simulink model "Electrical_System_2018b_obfs"  (R2019b)
settings: Solver=VariableStepAuto  StartTime=0.0  StopTime=5  RelTol=1e-3  AbsTol=1e-3  EnableMultiTasking=on
InitFcn:
  | Steady_State_Initialisation;
StopFcn:
  | %sscexplore(simlog);
  | %Logging
undefined symbols (not defined in the file): abrlhklxvp, aexgmhuedq, afmfmjnutg, afpphrjpnc, ahuxbyvruc, alarvljztt, amxnyqmnuw, aodrlwvqie, aolhmuplyq, aqpmguuqkg, auesgwirzl, aurophlnng, awamelrhru, ayfhvxflxn, azxkacuhqc, babszerikg, bawhdqanwq, bevoqecvei, bltjvqbchx, bmqsuewujl, bsmyqjfgnf, btvjbsmnve, bywgxqeadw, bziaduxaer, bzmcmdqocb, bzsvyvetat, ccsjnrbsih, cdvenygxwh, cedkrnslhx, cjheorclzs, cjrdshrtqx, ckhavyhcza, ckxewznhlz, cmrcgyiplk, conenicnws, cqkejbgjnn, csfnuwymhe, cunupkhwbh, cwzfvzuxxh, dcadmadufn, dcfponivnv, ddtrqjrhjn, dfhoxvkqas, dfrhtcwpne, dfvomcagjv, djijwylxea, dnmeqksrrm, dnzewbdkaa, dsqcykyxav, dtswwlttmm, ecumpidjtv, edegaywrct, ejjjsmnejc, eknqnehjdz, emvdetzouf, esxbqkbahr, etnkkbreiq, eunoiiiirw, ewewcuedir, fatkfxdhtc ... (+386)
libraries: fl_lib x802, ee_lib x362, fl_ps_legacy_lib x160, nesl_utility x85
(part 7 of 26)

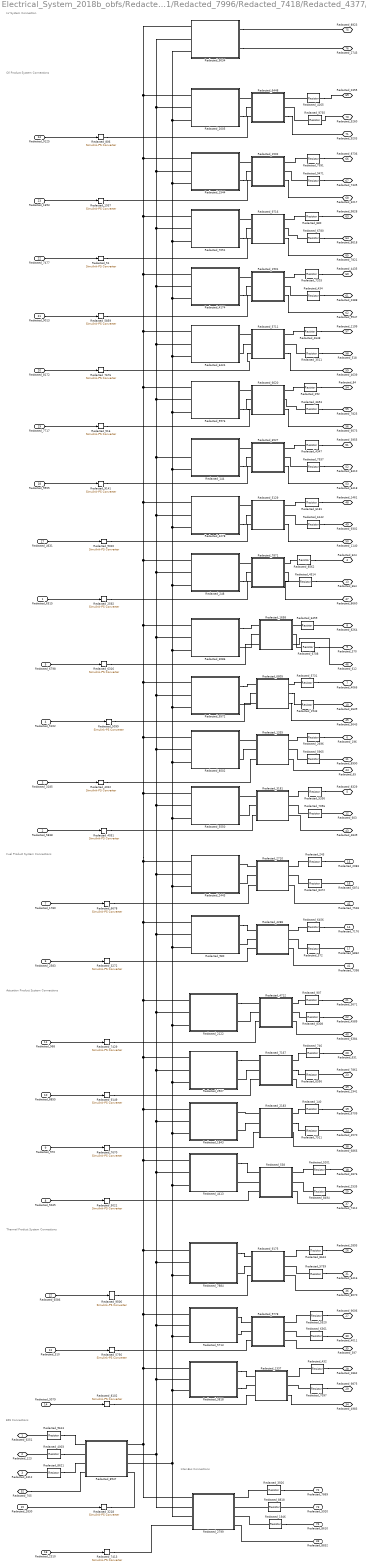
== system Electrical_System_2018b_obfs/Redacted_1221/Redacted_7996/Redacted_7418/Redacted_4377/Redacted_6082 ==
  note: LV System Connection
  note: Oil Product System Connections
  note: Fuel Product System Connections
  note: Actuation Product System Connections
  note: Thermal Product System Connections
  note: Inter-Bus Connections
  note: ESS Connections
  Redacted_6515 : Inport
  Redacted_5838 : Inport  Port=2
  Redacted_3185 : Inport  Port=3
  Redacted_5102 : Inport  Port=4
  Redacted_6798 : Inport  Port=5
  Redacted_2583 : Inport  Port=6
  Redacted_1780 : Inport  Port=7
  Redacted_5045 : Inport  Port=8
  Redacted_970 : Inport  Port=9
  Redacted_8855 : Inport  Port=10
  Redacted_968 : Inport  Port=11
  Redacted_6586 : Inport  Port=12
  Redacted_310 : Inport  Port=13
  Redacted_3079 : Inport  Port=14
  Redacted_2830 : Inport  Port=15
  Redacted_2310 : Inport  Port=16
  Redacted_4631 : Inport  Port=17
  Redacted_9555 : Inport  Port=18
  Redacted_7717 : Inport  Port=19
  Redacted_8172 : Inport  Port=20
  Redacted_9013 : Inport  Port=21
  Redacted_7477 : Inport  Port=22
  Redacted_1693 : Inport  Port=23
  Redacted_9125 : Inport  Port=24
  Redacted_1335 : Subsystem
      mask Display: image('SSPC.PNG'); % Use "Edit Image" on toolstrip to change.
  Redacted_1337 : Subsystem
      mask Display: image('SSPC.PNG'); % Use "Edit Image" on toolstrip to change.
  Redacted_140 : fl_lib/Electrical/Electrical Elements/Resistor  R=bywgxqeadw Ohm  i_specify=off  i_priority=None  i=aaernzfttg A  i_nominal_specify=off  i_nominal_unit=A  i_nominal_value=qebrwdmvxi  v_specify=off  v_priority=None  v=lmcajldehk V  v_nominal_specify=off  v_nominal_unit=V  v_nominal_value=linaoyeqjr
  Redacted_144 : Subsystem  VariantControlMode=Label  Variant=on  VariantControl=Variant1  LabelModeActiveChoice=Variant2
      mask Display: image('Rail Connection.png'); % Use "Edit Image" on toolstrip to change.
  Redacted_1502 : Subsystem
      mask Display: image('SSPC.PNG'); % Use "Edit Image" on toolstrip to change.
  Redacted_1544 : Subsystem  VariantControlMode=Label  Variant=on  VariantControl=Variant1  LabelModeActiveChoice=Variant2
      mask Display: image('Rail Connection.png'); % Use "Edit Image" on toolstrip to change.
  Redacted_1658 : Subsystem
      mask Display: image('SSPC.PNG'); % Use "Edit Image" on toolstrip to change.
  Redacted_1843 : Subsystem  VariantControlMode=Label  Variant=on  VariantControl=Variant1  LabelModeActiveChoice=Variant2
      mask Display: image('Rail Connection.png'); % Use "Edit Image" on toolstrip to change.
  Redacted_1901 : Subsystem
      mask Display: image('SSPC.PNG'); % Use "Edit Image" on toolstrip to change.
  Redacted_{51,516,806,1937,2592,3218,3272,4022,4051,5021,5099,5756,5859,6316,6678,7413,7429,7670,7676,8102,9020,9141,9149,9506} (24 alike) : nesl_utility/Simulink-PS Converter  PhysicalDomain=network_engine_domain  SubClassName=ps_input  LeftPortType=input  RightPortType=output  PseudoPeriodic=off  Frequencies=[]  NoiseDistribution=none  NoiseParameters=[]  Unit=1  AffineConversion=off  FilteringAndDerivatives=provide  SimscapeFilterOrder=1  InputFilterTimeConstant=0.001  UdotUserProvided=0
  Redacted_1943 : fl_lib/Electrical/Electrical Elements/Resistor  R=udeugimook Ohm  i_specify=off  i_priority=None  i=puzwctfirb A  i_nominal_specify=off  i_nominal_unit=A  i_nominal_value=umkambvvqu  v_specify=off  v_priority=None  v=urrixpqndl V  v_nominal_specify=off  v_nominal_unit=V  v_nominal_value=whwjtjekag
  Redacted_1946 : fl_lib/Electrical/Electrical Elements/Resistor  R=mqmlaotmlj Ohm  i_specify=off  i_priority=None  i=gywvblnqpy A  i_nominal_specify=off  i_nominal_unit=A  i_nominal_value=cimwjkbyvc  v_specify=off  v_priority=None  v=vgrxmuqnaa V  v_nominal_specify=off  v_nominal_unit=V  v_nominal_value=plxrtwzary
  Redacted_2005 : Subsystem  VariantControlMode=Label  Variant=on  VariantControl=Variant1  LabelModeActiveChoice=Variant2
      mask Display: image('Rail Connection.png'); % Use "Edit Image" on toolstrip to change.
  Redacted_2122 : Subsystem  VariantControlMode=Label  Variant=on  VariantControl=Variant1  LabelModeActiveChoice=Variant2
      mask Display: image('Rail Connection.png'); % Use "Edit Image" on toolstrip to change.
  Redacted_2183 : Subsystem
      mask Display: image('SSPC.PNG'); % Use "Edit Image" on toolstrip to change.
  Redacted_243 : fl_lib/Electrical/Electrical Elements/Resistor  R=qigyojbsct Ohm  i_specify=off  i_priority=None  i=cmdkiqythe A  i_nominal_specify=off  i_nominal_unit=A  i_nominal_value=bgvrsuqkke  v_specify=off  v_priority=None  v=requdmgyje V  v_nominal_specify=off  v_nominal_unit=V  v_nominal_value=wmmnzganav
  Redacted_2443 : Subsystem  VariantControlMode=Label  Variant=on  VariantControl=Variant1  LabelModeActiveChoice=Variant2
      mask Display: image('Rail Connection.png'); % Use "Edit Image" on toolstrip to change.
  Redacted_248 : Subsystem  VariantControlMode=Label  Variant=on  VariantControl=Variant1  LabelModeActiveChoice=Variant2
      mask Display: image('Rail Connection.png'); % Use "Edit Image" on toolstrip to change.
  Redacted_2696 : fl_lib/Electrical/Electrical Elements/Resistor  R=mcplwagmyk Ohm  i_specify=off  i_priority=None  i=aclovukjjc A  i_nominal_specify=off  i_nominal_unit=A  i_nominal_value=sujbwtvvoo  v_specify=off  v_priority=None  v=txlgwgsyxf V  v_nominal_specify=off  v_nominal_unit=V  v_nominal_value=xpmnlivytg
  Redacted_2710 : Subsystem
      mask Display: image('SSPC.PNG'); % Use "Edit Image" on toolstrip to change.
  Redacted_2799 : Subsystem
      mask Display: image('SSPC.PNG'); % Use "Edit Image" on toolstrip to change.
  Redacted_292 : fl_lib/Electrical/Electrical Elements/Resistor  R=menauypgpo Ohm  i_specify=off  i_priority=None  i=wfosbgtiga A  i_nominal_specify=off  i_nominal_unit=A  i_nominal_value=ekdspgvrvp  v_specify=off  v_priority=None  v=yxxjraphsi V  v_nominal_specify=off  v_nominal_unit=V  v_nominal_value=fepttdgqiv
  Redacted_2927 : Subsystem  VariantControlMode=Label  Variant=on  VariantControl=Variant1  LabelModeActiveChoice=Variant2
      mask Display: image('Rail Connection.png'); % Use "Edit Image" on toolstrip to change.
  Redacted_3086 : Subsystem  VariantControlMode=Label  Variant=on  VariantControl=Variant1  LabelModeActiveChoice=Variant2
      mask Display: image('Rail Connection.png'); % Use "Edit Image" on toolstrip to change.
  Redacted_3181 : Subsystem
      mask Display: image('SSPC.PNG'); % Use "Edit Image" on toolstrip to change.
  Redacted_3511 : fl_lib/Electrical/Electrical Elements/Resistor  R=ylisyynixv Ohm  i_specify=off  i_priority=None  i=ffgrnqlucb A  i_nominal_specify=off  i_nominal_unit=A  i_nominal_value=ftznbinimd  v_specify=off  v_priority=None  v=svytkptrjb V  v_nominal_specify=off  v_nominal_unit=V  v_nominal_value=jqejiqgqyo
  Redacted_3653 : fl_lib/Electrical/Electrical Elements/Resistor  R=xgtzgtozjh Ohm  i_specify=off  i_priority=None  i=jnxbdbomdp A  i_nominal_specify=off  i_nominal_unit=A  i_nominal_value=gzaofvhzxg  v_specify=off  v_priority=None  v=iuwoiyozby V  v_nominal_specify=off  v_nominal_unit=V  v_nominal_value=kxuhzkhadt
  Redacted_372 : fl_lib/Electrical/Electrical Elements/Resistor  R=auesgwirzl Ohm  i_specify=off  i_priority=None  i=uztwiwrozr A  i_nominal_specify=off  i_nominal_unit=A  i_nominal_value=hvaznjhdov  v_specify=off  v_priority=None  v=srejsyqirc V  v_nominal_specify=off  v_nominal_unit=V  v_nominal_value=aeuxvewjrt
  Redacted_3818 : Subsystem  VariantControlMode=Label  Variant=on  VariantControl=Variant1  LabelModeActiveChoice=Variant2
      mask Display: image('Rail Connection.png'); % Use "Edit Image" on toolstrip to change.
  Redacted_3926 : fl_lib/Electrical/Electrical Elements/Resistor  R=nxlhepldkb Ohm  i_specify=off  i_priority=None  i=eebivagpwk A  i_nominal_specify=off  i_nominal_unit=A  i_nominal_value=fufozlnnxg  v_specify=off  v_priority=None  v=dtlxktaynb V  v_nominal_specify=off  v_nominal_unit=V  v_nominal_value=dszddrzkvx
  Redacted_4003 : fl_lib/Electrical/Electrical Elements/Resistor  R=vrnsbvacfe Ohm  i_specify=off  i_priority=None  i=gvbuhntsho A  i_nominal_specify=off  i_nominal_unit=A  i_nominal_value=munqyifjoh  v_specify=off  v_priority=None  v=jbyfstdpct V  v_nominal_specify=off  v_nominal_unit=V  v_nominal_value=mnlizwupgn
  Redacted_4174 : Subsystem  VariantControlMode=Label  Variant=on  VariantControl=Variant1  LabelModeActiveChoice=Variant2
      mask Display: image('Rail Connection.png'); % Use "Edit Image" on toolstrip to change.
  Redacted_4265 : fl_lib/Electrical/Electrical Elements/Resistor  R=gudzapjreb Ohm  i_specify=off  i_priority=None  i=obmkkszubb A  i_nominal_specify=off  i_nominal_unit=A  i_nominal_value=oalecffgmr  v_specify=off  v_priority=None  v=gxitftarts V  v_nominal_specify=off  v_nominal_unit=V  v_nominal_value=jjmvhkfveq
  Redacted_4278 : Subsystem  VariantControlMode=Label  Variant=on  VariantControl=Variant1  LabelModeActiveChoice=Variant2
      mask Display: image('Rail Connection.png'); % Use "Edit Image" on toolstrip to change.
  Redacted_4288 : Subsystem
      mask Display: image('SSPC.PNG'); % Use "Edit Image" on toolstrip to change.
  Redacted_432 : fl_lib/Electrical/Electrical Elements/Resistor  R=uriccjuoow Ohm  i_specify=off  i_priority=None  i=cjvpnluohv A  i_nominal_specify=off  i_nominal_unit=A  i_nominal_value=rcknrpcbhc  v_specify=off  v_priority=None  v=ylhthilukt V  v_nominal_specify=off  v_nominal_unit=V  v_nominal_value=qemspzxdnp
  Redacted_434 : fl_lib/Electrical/Electrical Elements/Resistor  R=vjlkklkqng Ohm  i_specify=off  i_priority=None  i=htrxmzxdtf A  i_nominal_specify=off  i_nominal_unit=A  i_nominal_value=vksnoslwly  v_specify=off  v_priority=None  v=dndljnsomo V  v_nominal_specify=off  v_nominal_unit=V  v_nominal_value=fxljqvkixb
  Redacted_4347 : fl_lib/Electrical/Electrical Elements/Resistor  R=plfvgzzwna Ohm  i_specify=off  i_priority=None  i=nbkmkvgpyn A  i_nominal_specify=off  i_nominal_unit=A  i_nominal_value=ioasmbbgbs  v_specify=off  v_priority=None  v=zqtfzmktkd V  v_nominal_specify=off  v_nominal_unit=V  v_nominal_value=pujletubho
  Redacted_4413 : Subsystem  VariantControlMode=Label  Variant=on  VariantControl=Variant1  LabelModeActiveChoice=Variant2
      mask Display: image('Rail Connection.png'); % Use "Edit Image" on toolstrip to change.
  Redacted_4514 : fl_lib/Electrical/Electrical Elements/Resistor  R=mmxdiauzok Ohm  i_specify=off  i_priority=None  i=vowuozumvi A  i_nominal_specify=off  i_nominal_unit=A  i_nominal_value=kpbplzdbkq  v_specify=off  v_priority=None  v=qerizbmzjb V  v_nominal_specify=off  v_nominal_unit=V  v_nominal_value=nxpyqtyomq
  Redacted_4648 : fl_lib/Electrical/Electrical Elements/Resistor  R=qexlqsmnvg Ohm  i_specify=off  i_priority=None  i=gnkikzibrj A  i_nominal_specify=off  i_nominal_unit=A  i_nominal_value=baleaudnpn  v_specify=off  v_priority=None  v=ffvylbenjm V  v_nominal_specify=off  v_nominal_unit=V  v_nominal_value=cfxpwinlqu
  Redacted_4712 : Subsystem
      mask Display: image('SSPC.PNG'); % Use "Edit Image" on toolstrip to change.
  Redacted_5129 : Subsystem
      mask Display: image('SSPC.PNG'); % Use "Edit Image" on toolstrip to change.
  Redacted_5201 : fl_lib/Electrical/Electrical Elements/Resistor  R=zzyolnrdfp Ohm  i_specify=off  i_priority=None  i=vkqlttdaxe A  i_nominal_specify=off  i_nominal_unit=A  i_nominal_value=jbgufyqiak  v_specify=off  v_priority=None  v=ryvulvakfc V  v_nominal_specify=off  v_nominal_unit=V  v_nominal_value=rrrdmwanut
  Redacted_5336 : fl_lib/Electrical/Electrical Elements/Resistor  R=nryuhopuox Ohm  i_specify=off  i_priority=None  i=htkgszbxst A  i_nominal_specify=off  i_nominal_unit=A  i_nominal_value=eglwvqygkt  v_specify=off  v_priority=None  v=hqfgifczwz V  v_nominal_specify=off  v_nominal_unit=V  v_nominal_value=tsbftjsfcl
  Redacted_538 : Subsystem
      mask Display: image('SSPC.PNG'); % Use "Edit Image" on toolstrip to change.
  Redacted_5520 : fl_lib/Electrical/Electrical Elements/Resistor  R=skzfaryxlf Ohm  i_specify=off  i_priority=None  i=wzbtqjuhlr A  i_nominal_specify=off  i_nominal_unit=A  i_nominal_value=fgncuqysvt  v_specify=off  v_priority=None  v=cbggedjurd V  v_nominal_specify=off  v_nominal_unit=V  v_nominal_value=rojgpowexk
  Redacted_5550 : Subsystem  VariantControlMode=Label  Variant=on  VariantControl=Variant1  LabelModeActiveChoice=Variant2
      mask Display: image('Rail Connection.png'); % Use "Edit Image" on toolstrip to change.
  Redacted_5711 : Subsystem
      mask Display: image('SSPC.PNG'); % Use "Edit Image" on toolstrip to change.
  Redacted_5713 : Subsystem  VariantControlMode=Label  Variant=on  VariantControl=Variant1  LabelModeActiveChoice=Variant2
      mask Display: image('Rail Connection.png'); % Use "Edit Image" on toolstrip to change.
  Redacted_5731 : fl_lib/Electrical/Electrical Elements/Resistor  R=rnnynvlflh Ohm  i_specify=off  i_priority=None  i=gbmkfdxdgc A  i_nominal_specify=off  i_nominal_unit=A  i_nominal_value=pwtbhfeqep  v_specify=off  v_priority=None  v=nmvxveyulc V  v_nominal_specify=off  v_nominal_unit=V  v_nominal_value=hmwyzykwvo
  Redacted_5759 : fl_lib/Electrical/Electrical Elements/Resistor  R=omjgorwhkk Ohm  i_specify=off  i_priority=None  i=hwlgjrawps A  i_nominal_specify=off  i_nominal_unit=A  i_nominal_value=iyjrhrkuat  v_specify=off  v_priority=None  v=ebtsvlnfua V  v_nominal_specify=off  v_nominal_unit=V  v_nominal_value=vttgqnkzys
  Redacted_5965 : fl_lib/Electrical/Electrical Elements/Resistor  R=urgvbluqrp Ohm  i_specify=off  i_priority=None  i=sdpuusfedt A  i_nominal_specify=off  i_nominal_unit=A  i_nominal_value=ainxwvktfk  v_specify=off  v_priority=None  v=nvxgaiewlz V  v_nominal_specify=off  v_nominal_unit=V  v_nominal_value=ajceozfwvj
  Redacted_5976 : Subsystem  VariantControlMode=Label  Variant=on  VariantControl=Variant1  LabelModeActiveChoice=Variant2
      mask Display: image('Rail Connection.png'); % Use "Edit Image" on toolstrip to change.
  Redacted_6142 : fl_lib/Electrical/Electrical Elements/Resistor  R=mncmdqigre Ohm  i_specify=off  i_priority=None  i=wqwjalngmy A  i_nominal_specify=off  i_nominal_unit=A  i_nominal_value=nztynkvicp  v_specify=off  v_priority=None  v=idmlibbrmr V  v_nominal_specify=off  v_nominal_unit=V  v_nominal_value=jvxqddqmfb
  Redacted_6181 : fl_lib/Electrical/Electrical Elements/Resistor  R=fqkzdgzsgu Ohm  i_specify=off  i_priority=None  i=fnzwbqkjap A  i_nominal_specify=off  i_nominal_unit=A  i_nominal_value=esldlindrr  v_specify=off  v_priority=None  v=vccirnlvmw V  v_nominal_specify=off  v_nominal_unit=V  v_nominal_value=dsnehswwfw
  Redacted_6361 : fl_lib/Electrical/Electrical Elements/Resistor  R=ovtbszsvzf Ohm  i_specify=off  i_priority=None  i=jfnsuwlxbu A  i_nominal_specify=off  i_nominal_unit=A  i_nominal_value=sbvgbshvrr  v_specify=off  v_priority=None  v=vqnybtmmiq V  v_nominal_specify=off  v_nominal_unit=V  v_nominal_value=pwmsztivdy
  Redacted_6424 : Subsystem  VariantControlMode=Label  Variant=on  VariantControl=Variant1  LabelModeActiveChoice=Variant2
      mask Display: image('Rail Connection.png'); % Use "Edit Image" on toolstrip to change.
  Redacted_6448 : Subsystem
      mask Display: image('SSPC.PNG'); % Use "Edit Image" on toolstrip to change.
  Redacted_6456 : fl_lib/Electrical/Electrical Elements/Resistor  R=tusbxbupgx Ohm  i_specify=off  i_priority=None  i=rrbmtkstto A  i_nominal_specify=off  i_nominal_unit=A  i_nominal_value=khkvlwkofl  v_specify=off  v_priority=None  v=qiuodajtrd V  v_nominal_specify=off  v_nominal_unit=V  v_nominal_value=ejflqkzsax
  Redacted_6459 : fl_lib/Electrical/Electrical Elements/Resistor  R=cqkejbgjnn Ohm  i_specify=off  i_priority=None  i=tbwjgcwxqn A  i_nominal_specify=off  i_nominal_unit=A  i_nominal_value=plyjveijzz  v_specify=off  v_priority=None  v=weoewvqhjo V  v_nominal_specify=off  v_nominal_unit=V  v_nominal_value=ukqkdqpoud
  Redacted_6527 : Subsystem
      mask Display: image('SSPC.PNG'); % Use "Edit Image" on toolstrip to change.
  Redacted_6556 : fl_lib/Electrical/Electrical Elements/Resistor  R=fmwqrkuvkd Ohm  i_specify=off  i_priority=None  i=dwgmrctsil A  i_nominal_specify=off  i_nominal_unit=A  i_nominal_value=wijjhtyxqm  v_specify=off  v_priority=None  v=evictwdpah V  v_nominal_specify=off  v_nominal_unit=V  v_nominal_value=fqsaqtdnun
  Redacted_6620 : Subsystem
      mask Display: image('SSPC.PNG'); % Use "Edit Image" on toolstrip to change.
  Redacted_6708 : fl_lib/Electrical/Electrical Elements/Resistor  R=amxnyqmnuw Ohm  i_specify=off  i_priority=None  i=vfaufhwmjm A  i_nominal_specify=off  i_nominal_unit=A  i_nominal_value=tsznocxhec  v_specify=off  v_priority=None  v=qckytndsvg V  v_nominal_specify=off  v_nominal_unit=V  v_nominal_value=qxvgsujafj
  Redacted_6780 : fl_lib/Electrical/Electrical Elements/Resistor  R=mhdhhdazvr Ohm  i_specify=off  i_priority=None  i=tushcgsisj A  i_nominal_specify=off  i_nominal_unit=A  i_nominal_value=eiscctyztq  v_specify=off  v_priority=None  v=mvdkccfvee V  v_nominal_specify=off  v_nominal_unit=V  v_nominal_value=dfezcbrvkt
  Redacted_6805 : Subsystem
      mask Display: image('SSPC.PNG'); % Use "Edit Image" on toolstrip to change.
  Redacted_7051 : Subsystem  VariantControlMode=Label  Variant=on  VariantControl=Variant1  LabelModeActiveChoice=Variant2
      mask Display: image('Rail Connection.png'); % Use "Edit Image" on toolstrip to change.
  Redacted_7056 : fl_lib/Electrical/Electrical Elements/Resistor  R=cwzfvzuxxh Ohm  i_specify=off  i_priority=None  i=mfekpjbttp A  i_nominal_specify=off  i_nominal_unit=A  i_nominal_value=lbnrmtccgs  v_specify=off  v_priority=None  v=naoonpdaua V  v_nominal_specify=off  v_nominal_unit=V  v_nominal_value=dyqabnphiu
  Redacted_7097 : fl_lib/Electrical/Electrical Elements/Resistor  R=ccsjnrbsih Ohm  i_specify=off  i_priority=None  i=smlmepzbhs A  i_nominal_specify=off  i_nominal_unit=A  i_nominal_value=sahjpdtbbd  v_specify=off  v_priority=None  v=zanlnqweyo V  v_nominal_specify=off  v_nominal_unit=V  v_nominal_value=iuwykvtsqs
  Redacted_7167 : Subsystem
      mask Display: image('SSPC.PNG'); % Use "Edit Image" on toolstrip to change.
  Redacted_7203 : fl_lib/Electrical/Electrical Elements/Resistor  R=hvbuvcnqhj Ohm  i_specify=off  i_priority=None  i=evhpunisey A  i_nominal_specify=off  i_nominal_unit=A  i_nominal_value=xkumjsrtlw  v_specify=off  v_priority=None  v=froiuloxug V  v_nominal_specify=off  v_nominal_unit=V  v_nominal_value=qqirlwbqsg
  Redacted_746 : fl_lib/Electrical/Electrical Elements/Resistor  R=gyfrxmxkjw Ohm  i_specify=off  i_priority=None  i=kqwcsjfbhw A  i_nominal_specify=off  i_nominal_unit=A  i_nominal_value=uiiwupttxw  v_specify=off  v_priority=None  v=cmydbwsdof V  v_nominal_specify=off  v_nominal_unit=V  v_nominal_value=inycptujqr
  Redacted_7511 : fl_lib/Electrical/Electrical Elements/Resistor  R=xcokxmrlfm Ohm  i_specify=off  i_priority=None  i=mbghylsenz A  i_nominal_specify=off  i_nominal_unit=A  i_nominal_value=hutfywjieu  v_specify=off  v_priority=None  v=xdwiztyulb V  v_nominal_specify=off  v_nominal_unit=V  v_nominal_value=pkehylgvpr
  Redacted_7871 : Subsystem
      mask Display: image('SSPC.PNG'); % Use "Edit Image" on toolstrip to change.
  Redacted_7884 : Subsystem  VariantControlMode=Label  Variant=on  VariantControl=Variant1  LabelModeActiveChoice=Variant2
      mask Display: image('Rail Connection.png'); % Use "Edit Image" on toolstrip to change.
  Redacted_7937 : fl_lib/Electrical/Electrical Elements/Resistor  R=fvyxreljzk Ohm  i_specify=off  i_priority=None  i=xdhylptwsf A  i_nominal_specify=off  i_nominal_unit=A  i_nominal_value=zbydvhrhio  v_specify=off  v_priority=None  v=ezfcbzlgue V  v_nominal_specify=off  v_nominal_unit=V  v_nominal_value=ddpgvasxgz
  Redacted_7991 : fl_lib/Electrical/Electrical Elements/Resistor  R=ruienowprk Ohm  i_specify=off  i_priority=None  i=ctamepwubm A  i_nominal_specify=off  i_nominal_unit=A  i_nominal_value=qsikpskyme  v_specify=off  v_priority=None  v=xhyztbqbat V  v_nominal_specify=off  v_nominal_unit=V  v_nominal_value=dixnvpbgku
  Redacted_8308 : fl_lib/Electrical/Electrical Elements/Resistor  R=tiiudxdqfy Ohm  i_specify=off  i_priority=None  i=plpqkwaqfa A  i_nominal_specify=off  i_nominal_unit=A  i_nominal_value=arunkemdsp  v_specify=off  v_priority=None  v=fmpiezifcd V  v_nominal_specify=off  v_nominal_unit=V  v_nominal_value=bqqdvycabd
  Redacted_8472 : fl_lib/Electrical/Electrical Elements/Resistor  R=pfkbxapsma Ohm  i_specify=off  i_priority=None  i=vexbpfuymn A  i_nominal_specify=off  i_nominal_unit=A  i_nominal_value=aghpitybkl  v_specify=off  v_priority=None  v=kzsxozabsp V  v_nominal_specify=off  v_nominal_unit=V  v_nominal_value=ziprgcyfsh
  Redacted_8494 : fl_lib/Electrical/Electrical Elements/Resistor  R=fjreopucjn Ohm  i_specify=off  i_priority=None  i=ofxcooeske A  i_nominal_specify=off  i_nominal_unit=A  i_nominal_value=fairixoirf  v_specify=off  v_priority=None  v=xxugpzodlw V  v_nominal_specify=off  v_nominal_unit=V  v_nominal_value=vgnaxwehfe
  Redacted_8502 : Subsystem  VariantControlMode=Label  Variant=on  VariantControl=Variant1  LabelModeActiveChoice=Variant2
      mask Display: image('Rail Connection.png'); % Use "Edit Image" on toolstrip to change.
  Redacted_8562 : fl_lib/Electrical/Electrical Elements/Resistor  R=bziaduxaer Ohm  i_specify=off  i_priority=None  i=bcgstegszv A  i_nominal_specify=off  i_nominal_unit=A  i_nominal_value=luvqzyygsf  v_specify=off  v_priority=None  v=ipjpqqzwbl V  v_nominal_specify=off  v_nominal_unit=V  v_nominal_value=vfhnlwqrqj
  Redacted_8621 : fl_lib/Electrical/Electrical Elements/Resistor  R=vypdilqkfo Ohm  i_specify=off  i_priority=None  i=ylrnuvlfjb A  i_nominal_specify=off  i_nominal_unit=A  i_nominal_value=aolrdtjjum  v_specify=off  v_priority=None  v=jjszbjprpg V  v_nominal_specify=off  v_nominal_unit=V  v_nominal_value=glgregspev
  Redacted_8643 : fl_lib/Electrical/Electrical Elements/Resistor  R=tsamfrgnas Ohm  i_specify=off  i_priority=None  i=wfwveuunkx A  i_nominal_specify=off  i_nominal_unit=A  i_nominal_value=dxiwyduczd  v_specify=off  v_priority=None  v=ftptkdphjz V  v_nominal_specify=off  v_nominal_unit=V  v_nominal_value=epyvgbpebu
  Redacted_880 : fl_lib/Electrical/Electrical Elements/Resistor  R=jdehceuvmo Ohm  i_specify=off  i_priority=None  i=kqoqwmrfgc A  i_nominal_specify=off  i_nominal_unit=A  i_nominal_value=mbrmvtlznq  v_specify=off  v_priority=None  v=qovviumbhu V  v_nominal_specify=off  v_nominal_unit=V  v_nominal_value=erksdjajog
  Redacted_8818 : fl_lib/Electrical/Electrical Elements/Resistor  R=umtntjemde Ohm  i_specify=off  i_priority=None  i=uiznfwzliu A  i_nominal_specify=off  i_nominal_unit=A  i_nominal_value=tbwlsoqpbj  v_specify=off  v_priority=None  v=zsizmlginz V  v_nominal_specify=off  v_nominal_unit=V  v_nominal_value=jpqakujmjr
  Redacted_8947 : Subsystem
      mask Display: image('SSPC.PNG'); % Use "Edit Image" on toolstrip to change.
  Redacted_9034 : Subsystem  VariantControlMode=Label  Variant=on  VariantControl=Variant1  LabelModeActiveChoice=Variant2
      mask Display: image('Rail Connection.png'); % Use "Edit Image" on toolstrip to change.
  Redacted_907 : fl_lib/Electrical/Electrical Elements/Resistor  R=nthcrvjcbs Ohm  i_specify=off  i_priority=None  i=dhludlztrc A  i_nominal_specify=off  i_nominal_unit=A  i_nominal_value=axaxracutr  v_specify=off  v_priority=None  v=daqwyoxupm V  v_nominal_specify=off  v_nominal_unit=V  v_nominal_value=jrniddcjld
  Redacted_9175 : Subsystem
      mask Display: image('SSPC.PNG'); % Use "Edit Image" on toolstrip to change.
  Redacted_9471 : fl_lib/Electrical/Electrical Elements/Resistor  R=hajcebhcwj Ohm  i_specify=off  i_priority=None  i=etrpvgszev A  i_nominal_specify=off  i_nominal_unit=A  i_nominal_value=retbfkrjpe  v_specify=off  v_priority=None  v=wrbaggijzu V  v_nominal_specify=off  v_nominal_unit=V  v_nominal_value=iyktrdzodd
  Redacted_9572 : Subsystem  VariantControlMode=Label  Variant=on  VariantControl=Variant1  LabelModeActiveChoice=Variant2
      mask Display: image('Rail Connection.png'); % Use "Edit Image" on toolstrip to change.
  Redacted_9613 : fl_lib/Electrical/Electrical Elements/Resistor  R=npqbznhpbs Ohm  i_specify=off  i_priority=None  i=eqydrsehfi A  i_nominal_specify=off  i_nominal_unit=A  i_nominal_value=nndldggkyi  v_specify=off  v_priority=None  v=zicmjludhl V  v_nominal_specify=off  v_nominal_unit=V  v_nominal_value=qnjcqxjkyt
  Redacted_9716 : Subsystem
      mask Display: image('SSPC.PNG'); % Use "Edit Image" on toolstrip to change.
  Redacted_9735 : fl_lib/Electrical/Electrical Elements/Resistor  R=negsqlicnn Ohm  i_specify=off  i_priority=None  i=katqkzgarz A  i_nominal_specify=off  i_nominal_unit=A  i_nominal_value=oozoxszxgr  v_specify=off  v_priority=None  v=dfrexerunm V  v_nominal_specify=off  v_nominal_unit=V  v_nominal_value=oahkwowbas
  Redacted_9778 : Subsystem
      mask Display: image('SSPC.PNG'); % Use "Edit Image" on toolstrip to change.
  Redacted_980 : Subsystem  VariantControlMode=Label  Variant=on  VariantControl=Variant1  LabelModeActiveChoice=Variant2
      mask Display: image('Rail Connection.png'); % Use "Edit Image" on toolstrip to change.
  Redacted_9251 : PMIOPort  Side=Right
  Redacted_123 : PMIOPort  Port=2  Side=Right
  Redacted_4312 : PMIOPort  Port=3  Side=Right
  Redacted_624 : PMIOPort  Port=4  Side=Right
  Redacted_8329 : PMIOPort  Port=5  Side=Right
  Redacted_196 : PMIOPort  Port=6  Side=Right
  Redacted_4066 : PMIOPort  Port=7  Side=Right
  Redacted_8264 : PMIOPort  Port=8  Side=Right
  Redacted_370 : PMIOPort  Port=9  Side=Right
  Redacted_3639 : PMIOPort  Port=10  Side=Right
  Redacted_8990 : PMIOPort  Port=11  Side=Right
  Redacted_603 : PMIOPort  Port=12  Side=Right
  Redacted_664 : PMIOPort  Port=13  Side=Right
  Redacted_7176 : PMIOPort  Port=14  Side=Right
  Redacted_2083 : PMIOPort  Port=15  Side=Right
  Redacted_6874 : PMIOPort  Port=16  Side=Right
  Redacted_6862 : PMIOPort  Port=17  Side=Right
  Redacted_4876 : PMIOPort  Port=18  Side=Right
  Redacted_6709 : PMIOPort  Port=19  Side=Right
  Redacted_631 : PMIOPort  Port=20  Side=Right
  Redacted_3671 : PMIOPort  Port=21  Side=Right
  Redacted_4589 : PMIOPort  Port=22  Side=Right
  Redacted_7861 : PMIOPort  Port=23  Side=Right
  Redacted_4570 : PMIOPort  Port=24  Side=Right
  Redacted_2535 : PMIOPort  Port=25  Side=Right
  Redacted_2893 : PMIOPort  Port=26  Side=Right
  Redacted_9606 : PMIOPort  Port=27  Side=Right
  Redacted_1862 : PMIOPort  Port=28  Side=Right
  Redacted_9875 : PMIOPort  Port=29  Side=Right
  Redacted_4011 : PMIOPort  Port=30  Side=Right
  Redacted_6416 : PMIOPort  Port=31  Side=Right
  Redacted_705 : PMIOPort  Port=32  Side=Left
  Redacted_8832 : PMIOPort  Port=33  Side=Left
  Redacted_4983 : PMIOPort  Port=34  Side=Left
  Redacted_397 : PMIOPort  Port=35  Side=Left
  Redacted_8070 : PMIOPort  Port=36  Side=Left
  Redacted_7312 : PMIOPort  Port=37  Side=Left
  Redacted_6866 : PMIOPort  Port=38  Side=Left
  Redacted_1941 : PMIOPort  Port=39  Side=Left
  Redacted_6384 : PMIOPort  Port=40  Side=Left
  Redacted_7398 : PMIOPort  Port=41  Side=Left
  Redacted_7548 : PMIOPort  Port=42  Side=Left
  Redacted_4849 : PMIOPort  Port=43  Side=Left
  Redacted_65 : PMIOPort  Port=44  Side=Left
  Redacted_5643 : PMIOPort  Port=45  Side=Left
  Redacted_612 : PMIOPort  Port=46  Side=Left
  Redacted_8660 : PMIOPort  Port=47  Side=Left
  Redacted_1461 : PMIOPort  Port=48  Side=Right
  Redacted_9302 : PMIOPort  Port=49  Side=Right
  Redacted_1140 : PMIOPort  Port=50  Side=Left
  Redacted_3955 : PMIOPort  Port=51  Side=Right
  Redacted_8410 : PMIOPort  Port=52  Side=Right
  Redacted_6418 : PMIOPort  Port=53  Side=Left
  Redacted_84 : PMIOPort  Port=54  Side=Right
  Redacted_7825 : PMIOPort  Port=55  Side=Right
  Redacted_9573 : PMIOPort  Port=56  Side=Left
  Redacted_1199 : PMIOPort  Port=57  Side=Right
  Redacted_518 : PMIOPort  Port=58  Side=Right
  Redacted_4639 : PMIOPort  Port=59  Side=Left
  Redacted_4435 : PMIOPort  Port=60  Side=Right
  Redacted_2388 : PMIOPort  Port=61  Side=Right
  Redacted_9547 : PMIOPort  Port=62  Side=Left
  Redacted_9828 : PMIOPort  Port=63  Side=Right
  Redacted_8618 : PMIOPort  Port=64  Side=Right
  Redacted_7821 : PMIOPort  Port=65  Side=Left
  Redacted_8736 : PMIOPort  Port=66  Side=Right
  Redacted_7335 : PMIOPort  Port=67  Side=Right
  Redacted_3217 : PMIOPort  Port=68  Side=Left
  Redacted_2355 : PMIOPort  Port=69  Side=Right
  Redacted_5260 : PMIOPort  Port=70  Side=Right
  Redacted_9203 : PMIOPort  Port=71  Side=Left
  Redacted_7869 : PMIOPort  Port=72  Side=Right
  Redacted_5920 : PMIOPort  Port=73  Side=Right
  Redacted_8610 : PMIOPort  Port=74  Side=Right
  Redacted_8923 : PMIOPort  Port=75  Side=Right
  Redacted_2743 : PMIOPort  Port=76  Side=Right
  wires:
  Redacted_6586/1 -> Redacted_9506/1
  Redacted_3079/1 -> Redacted_8102/1
  Redacted_2310/1 -> Redacted_7413/1
  Redacted_2830/1 -> Redacted_3218/1
  Redacted_310/1 -> Redacted_5756/1
  Redacted_968/1 -> Redacted_7429/1
  Redacted_8855/1 -> Redacted_9149/1
  Redacted_970/1 -> Redacted_7670/1
  Redacted_5045/1 -> Redacted_5021/1
  Redacted_1780/1 -> Redacted_6678/1
  Redacted_2583/1 -> Redacted_3272/1
  Redacted_6798/1 -> Redacted_6316/1
  Redacted_5102/1 -> Redacted_5099/1
  Redacted_3185/1 -> Redacted_4022/1
  Redacted_5838/1 -> Redacted_4051/1
  Redacted_6515/1 -> Redacted_2592/1
  Redacted_4631/1 -> Redacted_9020/1
  Redacted_7717/1 -> Redacted_516/1
  Redacted_9555/1 -> Redacted_9141/1
  Redacted_7477/1 -> Redacted_51/1
  Redacted_1693/1 -> Redacted_1937/1
  Redacted_9013/1 -> Redacted_5859/1
  Redacted_8172/1 -> Redacted_7676/1
  Redacted_9125/1 -> Redacted_806/1
  connections:
  Redacted_3818/RConn1 -- Redacted_1337/RConn1
  Redacted_432/LConn1 -- Redacted_1337/LConn1
  Redacted_8102/RConn1 -- Redacted_1337/RConn3
  Redacted_5756/RConn1 -- Redacted_9778/RConn3
  Redacted_5759/LConn1 -- Redacted_6416/RConn1
  Redacted_9506/RConn1 -- Redacted_9175/RConn3
  Redacted_603/RConn1 -- Redacted_7056/LConn1
  Redacted_8990/RConn1 -- Redacted_5965/LConn1
  Redacted_3639/RConn1 -- Redacted_1943/LConn1
  Redacted_6708/LConn1 -- Redacted_370/RConn1
  Redacted_2592/RConn1 -- Redacted_7871/RConn3
  Redacted_4051/RConn1 -- Redacted_3181/RConn3
  Redacted_4022/RConn1 -- Redacted_1335/RConn3
  Redacted_5099/RConn1 -- Redacted_6805/RConn3
  Redacted_6316/RConn1 -- Redacted_1658/RConn3
  Redacted_4514/LConn1 -- Redacted_664/RConn1
  Redacted_4288/RConn3 -- Redacted_3272/RConn1
  Redacted_6678/RConn1 -- Redacted_2710/RConn3
  Redacted_6874/RConn1 -- Redacted_8472/LConn1
  Redacted_6862/RConn1 -- Redacted_372/LConn1
  Redacted_538/RConn3 -- Redacted_5021/RConn1
  Redacted_2183/RConn3 -- Redacted_7670/RConn1
  Redacted_9149/RConn1 -- Redacted_7167/RConn3
  Redacted_7429/RConn1 -- Redacted_4712/RConn3
  Redacted_8308/LConn1 -- Redacted_4589/RConn1
  Redacted_8502/LConn1 -- Redacted_2443/LConn1 -- Redacted_8947/RConn1 -- Redacted_2799/RConn1 -- Redacted_3818/LConn1 -- Redacted_5713/LConn1 -- Redacted_7884/LConn1 -- Redacted_4413/LConn1 -- Redacted_1843/LConn1 -- Redacted_2927/LConn1 -- Redacted_2122/LConn1 -- Redacted_980/LConn1 -- Redacted_5550/LConn1 -- Redacted_9572/LConn1 -- Redacted_3086/LConn1 -- Redacted_248/LConn1 -- Redacted_4278/LConn1 -- Redacted_5976/LConn1 -- Redacted_6424/LConn1 -- Redacted_4174/LConn1 -- Redacted_7051/LConn1 -- Redacted_1544/LConn1 -- Redacted_9034/LConn1 -- Redacted_2005/LConn1
  Redacted_7861/RConn1 -- Redacted_6556/LConn1
  Redacted_4570/RConn1 -- Redacted_7511/LConn1
  Redacted_2535/RConn1 -- Redacted_8494/LConn1
  Redacted_8502/LConn3 -- Redacted_2443/LConn3 -- Redacted_2799/RConn3 -- Redacted_8947/RConn3 -- Redacted_3818/LConn3 -- Redacted_5713/LConn3 -- Redacted_7884/LConn3 -- Redacted_4413/LConn3 -- Redacted_1843/LConn3 -- Redacted_2927/LConn3 -- Redacted_2122/LConn3 -- Redacted_980/LConn3 -- Redacted_5550/LConn3 -- Redacted_9572/LConn3 -- Redacted_3086/LConn3 -- Redacted_248/LConn3 -- Redacted_4278/LConn3 -- Redacted_144/LConn3 -- Redacted_5976/LConn3 -- Redacted_6424/LConn3 -- Redacted_4174/LConn3 -- Redacted_7051/LConn3 -- Redacted_1544/LConn3 -- Redacted_9034/LConn3 -- Redacted_2005/LConn3
  Redacted_8502/LConn2 -- Redacted_2443/LConn2 -- Redacted_980/LConn2 -- Redacted_5713/LConn2 -- Redacted_3818/LConn2 -- Redacted_2799/RConn2 -- Redacted_8947/RConn2 -- Redacted_7884/LConn2 -- Redacted_4413/LConn2 -- Redacted_1843/LConn2 -- Redacted_2927/LConn2 -- Redacted_2122/LConn2 -- Redacted_5550/LConn2 -- Redacted_9572/LConn2 -- Redacted_3086/LConn2 -- Redacted_248/LConn2 -- Redacted_4278/LConn2 -- Redacted_144/LConn2 -- Redacted_5976/LConn2 -- Redacted_6424/LConn2 -- Redacted_4174/LConn2 -- Redacted_7051/LConn2 -- Redacted_1544/LConn2 -- Redacted_9034/LConn2 -- Redacted_2005/LConn2
  Redacted_1946/RConn1 -- Redacted_8610/RConn1
  Redacted_8818/LConn1 -- Redacted_2799/LConn2
  Redacted_3926/RConn1 -- Redacted_7869/RConn1
  Redacted_7413/RConn1 -- Redacted_2799/RConn4
  Redacted_3218/RConn1 -- Redacted_8947/RConn4
  Redacted_9613/LConn1 -- Redacted_8947/LConn1
  Redacted_4003/RConn1 -- Redacted_123/RConn1
  Redacted_8621/RConn1 -- Redacted_4312/RConn1
  Redacted_7097/LConn1 -- Redacted_9875/RConn1
  Redacted_6361/LConn1 -- Redacted_4011/RConn1
  Redacted_9613/RConn1 -- Redacted_9251/RConn1
  Redacted_4003/LConn1 -- Redacted_8947/LConn2
  Redacted_8621/LConn1 -- Redacted_8947/LConn3
  Redacted_1946/LConn1 -- Redacted_2799/LConn3
  Redacted_3926/LConn1 -- Redacted_2799/LConn1
  Redacted_5920/RConn1 -- Redacted_8818/RConn1
  Redacted_432/RConn1 -- Redacted_1862/RConn1
  Redacted_5520/RConn1 -- Redacted_9606/RConn1
  Redacted_5520/LConn1 -- Redacted_9778/LConn1
  Redacted_5713/RConn1 -- Redacted_9778/RConn1
  Redacted_8643/RConn1 -- Redacted_2893/RConn1
  Redacted_7884/RConn1 -- Redacted_9175/RConn1
  Redacted_8643/LConn1 -- Redacted_9175/LConn1
  Redacted_6456/RConn1 -- Redacted_7176/RConn1
  Redacted_980/RConn1 -- Redacted_4288/RConn1
  Redacted_6456/LConn1 -- Redacted_4288/LConn1
  Redacted_243/RConn1 -- Redacted_2083/RConn1
  Redacted_243/LConn1 -- Redacted_2710/LConn1
  Redacted_2710/RConn1 -- Redacted_2443/RConn1
  Redacted_907/RConn1 -- Redacted_3671/RConn1
  Redacted_907/LConn1 -- Redacted_4712/LConn1
  Redacted_2122/RConn1 -- Redacted_4712/RConn1
  Redacted_2927/RConn1 -- Redacted_7167/RConn1
  Redacted_746/LConn1 -- Redacted_7167/LConn1
  Redacted_746/RConn1 -- Redacted_631/RConn1
  Redacted_140/LConn1 -- Redacted_2183/LConn1
  Redacted_140/RConn1 -- Redacted_6709/RConn1
  Redacted_2183/RConn1 -- Redacted_1843/RConn1
  Redacted_4413/RConn1 -- Redacted_538/RConn1
  Redacted_5201/RConn1 -- Redacted_4876/RConn1
  Redacted_5201/LConn1 -- Redacted_538/LConn1
  Redacted_8562/RConn1 -- Redacted_624/RConn1
  Redacted_8562/LConn1 -- Redacted_7871/LConn1
  Redacted_7871/RConn1 -- Redacted_248/RConn1
  Redacted_6459/LConn1 -- Redacted_1658/LConn1
  Redacted_8264/RConn1 -- Redacted_6459/RConn1
  Redacted_5731/RConn1 -- Redacted_4066/RConn1
  Redacted_5731/LConn1 -- Redacted_6805/LConn1
  Redacted_9572/RConn1 -- Redacted_6805/RConn1
  Redacted_3181/RConn1 -- Redacted_5550/RConn1
  Redacted_5336/LConn1 -- Redacted_3181/LConn1
  Redacted_5336/RConn1 -- Redacted_8329/RConn1
  Redacted_1335/RConn1 -- Redacted_8502/RConn1
  Redacted_2696/LConn1 -- Redacted_1335/LConn1
  Redacted_2696/RConn1 -- Redacted_196/RConn1
  Redacted_705/RConn1 -- Redacted_8947/LConn4
  Redacted_8832/RConn1 -- Redacted_2799/LConn4
  Redacted_3818/RConn2 -- Redacted_1337/RConn2
  Redacted_7097/RConn1 -- Redacted_1337/LConn2
  Redacted_1337/LConn3 -- Redacted_4983/RConn1
  Redacted_9778/RConn2 -- Redacted_5713/RConn2
  Redacted_6361/RConn1 -- Redacted_9778/LConn2
  Redacted_397/RConn1 -- Redacted_9778/LConn3
  Redacted_9175/RConn2 -- Redacted_7884/RConn2
  Redacted_5759/RConn1 -- Redacted_9175/LConn2
  Redacted_8070/RConn1 -- Redacted_9175/LConn3
  Redacted_538/RConn2 -- Redacted_4413/RConn2
  Redacted_8494/RConn1 -- Redacted_538/LConn2
  Redacted_2183/LConn2 -- Redacted_7511/RConn1
  Redacted_2183/RConn2 -- Redacted_1843/RConn2
  Redacted_7312/RConn1 -- Redacted_538/LConn3
  Redacted_6866/RConn1 -- Redacted_2183/LConn3
  Redacted_7167/LConn2 -- Redacted_6556/RConn1
  Redacted_7167/RConn2 -- Redacted_2927/RConn2
  Redacted_1941/RConn1 -- Redacted_7167/LConn3
  Redacted_8308/RConn1 -- Redacted_4712/LConn2
  Redacted_4712/RConn2 -- Redacted_2122/RConn2
  Redacted_6384/RConn1 -- Redacted_4712/LConn3
  Redacted_2710/RConn2 -- Redacted_2443/RConn2
  Redacted_8472/RConn1 -- Redacted_2710/LConn2
  Redacted_4288/RConn2 -- Redacted_980/RConn2
  Redacted_372/RConn1 -- Redacted_4288/LConn2
  Redacted_7398/RConn1 -- Redacted_4288/LConn3
  Redacted_7548/RConn1 -- Redacted_2710/LConn3
  Redacted_3181/RConn2 -- Redacted_5550/RConn2
  Redacted_7056/RConn1 -- Redacted_3181/LConn2
  Redacted_4849/RConn1 -- Redacted_3181/LConn3
  Redacted_5965/RConn1 -- Redacted_1335/LConn2
  Redacted_1335/RConn2 -- Redacted_8502/RConn2
  Redacted_65/RConn1 -- Redacted_1335/LConn3
  Redacted_4514/RConn1 -- Redacted_7871/LConn2
  Redacted_7871/LConn3 -- Redacted_8660/RConn1
  Redacted_248/RConn2 -- Redacted_7871/RConn2
  Redacted_6708/RConn1 -- Redacted_1658/LConn2
  Redacted_612/RConn1 -- Redacted_1658/LConn3
  Redacted_6805/RConn2 -- Redacted_9572/RConn2
  Redacted_6805/LConn2 -- Redacted_1943/RConn1
  Redacted_6805/LConn3 -- Redacted_5643/RConn1
  Redacted_1658/RConn2 -- Redacted_3086/RConn2
  Redacted_3086/RConn1 -- Redacted_1658/RConn1
  Redacted_5129/LConn3 -- Redacted_1140/RConn1
  Redacted_4278/RConn2 -- Redacted_5129/RConn2
  Redacted_6181/RConn1 -- Redacted_1461/RConn1
  Redacted_6142/RConn1 -- Redacted_5129/LConn2
  Redacted_6142/LConn1 -- Redacted_9302/RConn1
  Redacted_9020/RConn1 -- Redacted_5129/RConn3
  Redacted_6181/LConn1 -- Redacted_5129/LConn1
  Redacted_5129/RConn1 -- Redacted_4278/RConn1
  Redacted_6620/RConn1 -- Redacted_5976/RConn1
  Redacted_3653/LConn1 -- Redacted_7825/RConn1
  Redacted_3653/RConn1 -- Redacted_6620/LConn2
  Redacted_292/RConn1 -- Redacted_84/RConn1
  Redacted_516/RConn1 -- Redacted_6620/RConn3
  Redacted_5976/RConn2 -- Redacted_6620/RConn2
  Redacted_6527/LConn3 -- Redacted_6418/RConn1
  Redacted_144/RConn2 -- Redacted_6527/RConn2
  Redacted_4347/RConn1 -- Redacted_3955/RConn1
  Redacted_7937/RConn1 -- Redacted_6527/LConn2
  Redacted_292/LConn1 -- Redacted_6620/LConn1
  Redacted_7937/LConn1 -- Redacted_8410/RConn1
  Redacted_6620/LConn3 -- Redacted_9573/RConn1
  Redacted_9141/RConn1 -- Redacted_6527/RConn3
  Redacted_4347/LConn1 -- Redacted_6527/LConn1
  Redacted_6527/RConn1 -- Redacted_144/RConn1
  Redacted_9716/RConn1 -- Redacted_7051/RConn1
  Redacted_1502/LConn3 -- Redacted_3217/RConn1
  Redacted_880/LConn1 -- Redacted_9716/LConn1
  Redacted_6780/LConn1 -- Redacted_8618/RConn1
  Redacted_7991/LConn1 -- Redacted_1502/LConn1
  Redacted_6780/RConn1 -- Redacted_9716/LConn2
  Redacted_880/RConn1 -- Redacted_9828/RConn1
  Redacted_7051/RConn2 -- Redacted_9716/RConn2
  Redacted_9716/LConn3 -- Redacted_7821/RConn1
  Redacted_51/RConn1 -- Redacted_9716/RConn3
  Redacted_1544/RConn2 -- Redacted_1502/RConn2
  Redacted_1937/RConn1 -- Redacted_1502/RConn3
  Redacted_7991/RConn1 -- Redacted_8736/RConn1
  Redacted_9471/RConn1 -- Redacted_1502/LConn2
  Redacted_1901/RConn1 -- Redacted_4174/RConn1
  Redacted_434/LConn1 -- Redacted_2388/RConn1
  Redacted_434/RConn1 -- Redacted_1901/LConn2
  Redacted_7203/RConn1 -- Redacted_4435/RConn1
  Redacted_5859/RConn1 -- Redacted_1901/RConn3
  Redacted_4174/RConn2 -- Redacted_1901/RConn2
  Redacted_5711/LConn3 -- Redacted_4639/RConn1
  Redacted_6424/RConn2 -- Redacted_5711/RConn2
  Redacted_1502/RConn1 -- Redacted_1544/RConn1
  Redacted_4648/RConn1 -- Redacted_1199/RConn1
  Redacted_3511/RConn1 -- Redacted_5711/LConn2
  Redacted_7203/LConn1 -- Redacted_1901/LConn1
  Redacted_3511/LConn1 -- Redacted_518/RConn1
  Redacted_1901/LConn3 -- Redacted_9547/RConn1
  Redacted_9471/LConn1 -- Redacted_7335/RConn1
  Redacted_7676/RConn1 -- Redacted_5711/RConn3
  Redacted_4648/LConn1 -- Redacted_5711/LConn1
  Redacted_5711/RConn1 -- Redacted_6424/RConn1
  Redacted_6448/RConn1 -- Redacted_2005/RConn1
  Redacted_9735/RConn1 -- Redacted_6448/LConn2
  Redacted_9735/LConn1 -- Redacted_5260/RConn1
  Redacted_806/RConn1 -- Redacted_6448/RConn3
  Redacted_4265/RConn1 -- Redacted_2355/RConn1
  Redacted_4265/LConn1 -- Redacted_6448/LConn1
  Redacted_6448/LConn3 -- Redacted_9203/RConn1
  Redacted_2005/RConn2 -- Redacted_6448/RConn2
  Redacted_9034/RConn1 -- Redacted_8923/RConn1
  Redacted_9034/RConn2 -- Redacted_2743/RConn1
